simulink model "propagator_mess"  (R2023b)
settings: Solver=VariableStepAuto  StartTime=0.0  StopTime=tf  RelTol=1e-10  AbsTol=1e-10
undefined symbols (not defined in the file or in its folder): mass, thrust, thrustingThreshold
libraries: vrlib x3, simulink x1, aerolibsatdyn x1, aerolibutil x1
settings Model: SimulationMode=rapid-accelerator  Creator=miqui  LastModifiedBy=miqui

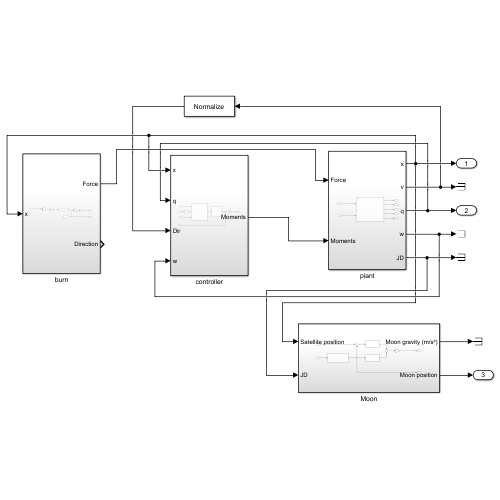
[thumbnail: Simulink's stored preview of the top-level diagram]
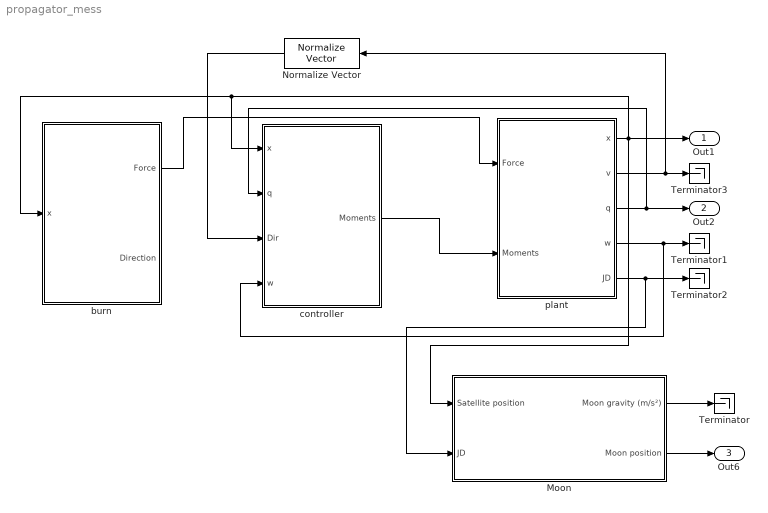
== system propagator_mess ==
  Moon : Subsystem
  Normalize Vector : vrlib/Utilities/Normalize Vector  maxzero=0
  Terminator{,1..3} (4 alike) : Terminator
  burn : Subsystem
  controller : Subsystem
  plant : Subsystem
  Out1 : Outport
  Out2 : Outport  Port=2
  Out6 : Outport  Port=3
  wires:
  plant/1(x) -> controller/1(x), burn/1(x), Moon/1(Satellite position), Out1/1
  plant/2(v) -> Normalize Vector/1, Terminator3/1
  plant/3(q) -> Out2/1, controller/2(q)
  plant/4(w) -> Terminator1/1, controller/4(w)
  plant/5(JD) -> Terminator2/1, Moon/2(JD)
  Moon/1(Moon gravity (m/s²)) -> Terminator/1
  Moon/2(Moon position) -> Out6/1
  Normalize Vector/1 -> controller/3(Dir)
  controller/1(Moments) -> plant/2(Moments)
  burn/1(Force) -> plant/1(Force)

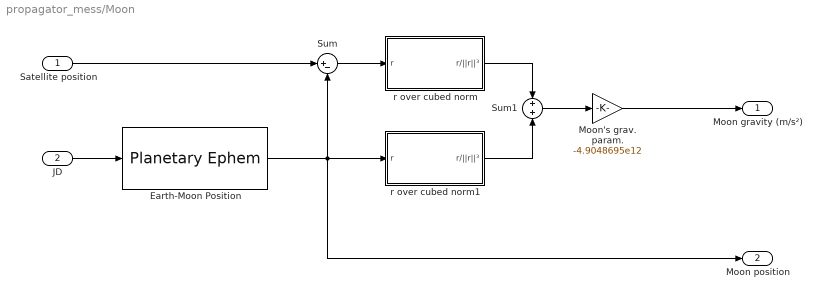
== system propagator_mess/Moon ==
  Satellite position : Inport
  JD : Inport  Port=2
  Earth-Moon Position : PlanetaryEphem  units=m,m/s  useDateRange=on  outputVelocity=off
  Moon's grav. param. : Gain  Gain=-4.9048695e12
  Sum : Sum  Inputs=|+-
  Sum1 : Sum
  r over cubed norm : Subsystem
  r over cubed norm1 : Subsystem
  Moon gravity (m/s²) : Outport
  Moon position : Outport  Port=2
  wires:
  JD/1 -> Earth-Moon Position/1
  Satellite position/1 -> Sum/1
  Earth-Moon Position/1 -> Moon position/1, r over cubed norm1/1(r), Sum/2
  Sum/1 -> r over cubed norm/1(r)
  Sum1/1 -> Moon's grav. param./1
  Moon's grav. param./1 -> Moon gravity (m/s²)/1
  r over cubed norm/1(r/||r||³) -> Sum1/1
  r over cubed norm1/1(r/||r||³) -> Sum1/2

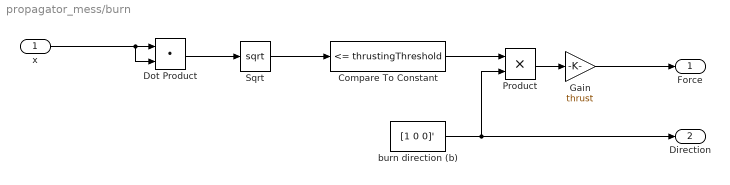
== system propagator_mess/burn ==
  x : Inport
  Compare To Constant : simulink/Logic and Bit Operations/Compare To Constant  relop=<=  const=thrustingThreshold  OutDataTypeStr=boolean
  Dot Product : DotProduct  OutDataTypeStr=Inherit: Inherit via internal rule
  Gain : Gain  Gain=thrust
  Product : Product
  Sqrt : Sqrt
  burn direction (b) : Constant  Value=[1 0 0]'
  Force : Outport
  Direction : Outport  Port=2
  wires:
  Dot Product/1 -> Sqrt/1
  Sqrt/1 -> Compare To Constant/1
  x/1 -> Dot Product/2, Dot Product/1
  burn direction (b)/1 -> Direction/1, Product/2
  Gain/1 -> Force/1
  Compare To Constant/1 -> Product/1
  Product/1 -> Gain/1

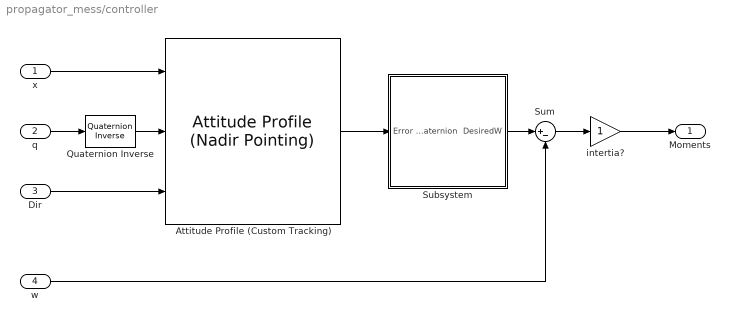
== system propagator_mess/controller ==
  x : Inport
  q : Inport  Port=2
  Dir : Inport  Port=3
  w : Inport  Port=4
  Attitude Profile (Custom Tracking) : aerolibsatdyn/Attitude Profile (Nadir Pointing)  outputError=on  outputFinalAttitude=off  portFrame=ICRF  pointingMode=Custom  celestialTarget=Sun  tunablePointing=off  primaryAlignmentSrc=Dialog  primaryAlignment=[1 0 0]  secondaryAlignmentSrc=Dialog  secondaryAlignment=[0 0 1]  constraintFrame=ICRF  primaryConstraintSrc=Port  primaryConstraint=[1 0 0]  secondaryConstraintSrc=Dialog  secondaryConstraint=[0 0 1]
      settings: LibrarySourceBlock=|
      | aerolibsatdyn/Attitude Profile
      | (Sun Tracking)
  Quaternion Inverse : aerolibutil/Quaternion Inverse
  Subsystem : Subsystem
  Sum : Sum  Inputs=|+-
  intertia? : Gain
  Moments : Outport
  wires:
  intertia?/1 -> Moments/1
  x/1 -> Attitude Profile (Custom Tracking)/1
  q/1 -> Quaternion Inverse/1
  Quaternion Inverse/1 -> Attitude Profile (Custom Tracking)/2
  Sum/1 -> intertia?/1
  w/1 -> Sum/2
  Attitude Profile (Custom Tracking)/1 -> Subsystem/1(Error quaternion)
  Subsystem/1(DesiredW) -> Sum/1
  Dir/1 -> Attitude Profile (Custom Tracking)/3

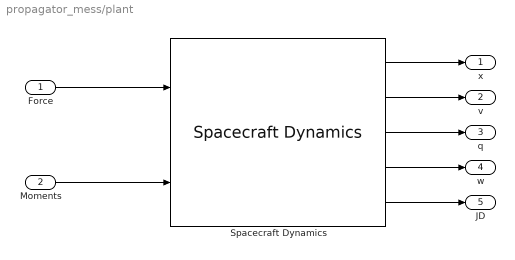
== system propagator_mess/plant ==
  Force : Inport
  Moments : Inport  Port=2
  Spacecraft Dynamics : SpacecraftDynamics  mass=mass  inertia=[1, 0, 0; 0, 1, 0; 0, 0, 1]*mass  useMassFlowRelativeVelocity=on  semiMajorAxis=sma  eccentricity=ecc  inclination=inc  raan=RAAN  argPeriapsis=aop  trueAnomaly=true_an  gravityModel=Point-mass  useEOPs=off
  x : Outport
  v : Outport  Port=2
  q : Outport  Port=3
  w : Outport  Port=4
  JD : Outport  Port=5
  wires:
  Spacecraft Dynamics/5 -> JD/1
  Spacecraft Dynamics/1 -> x/1
  Force/1 -> Spacecraft Dynamics/1
  Moments/1 -> Spacecraft Dynamics/2
  Spacecraft Dynamics/4 -> w/1
  Spacecraft Dynamics/2 -> v/1
  Spacecraft Dynamics/3 -> q/1

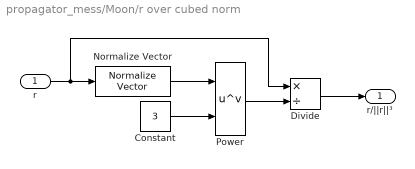
== system propagator_mess/Moon/r over cubed norm ==
  r : Inport
  Constant : Constant  Value=3
  Divide : Product  Inputs=*/
  Normalize Vector : vrlib/Utilities/Normalize Vector  maxzero=0
  Power : Math  Operator=pow
  r/||r||³ : Outport
  wires:
  r/1 -> Divide/1, Normalize Vector/1
  Normalize Vector/1 -> Power/1
  Constant/1 -> Power/2
  Power/1 -> Divide/2
  Divide/1 -> r/||r||³/1

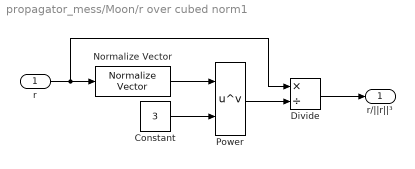
== system propagator_mess/Moon/r over cubed norm1 ==
  r : Inport
  Constant : Constant  Value=3
  Divide : Product  Inputs=*/
  Normalize Vector : vrlib/Utilities/Normalize Vector  maxzero=0
  Power : Math  Operator=pow
  r/||r||³ : Outport
  wires:
  r/1 -> Divide/1, Normalize Vector/1
  Normalize Vector/1 -> Power/1
  Constant/1 -> Power/2
  Power/1 -> Divide/2
  Divide/1 -> r/||r||³/1

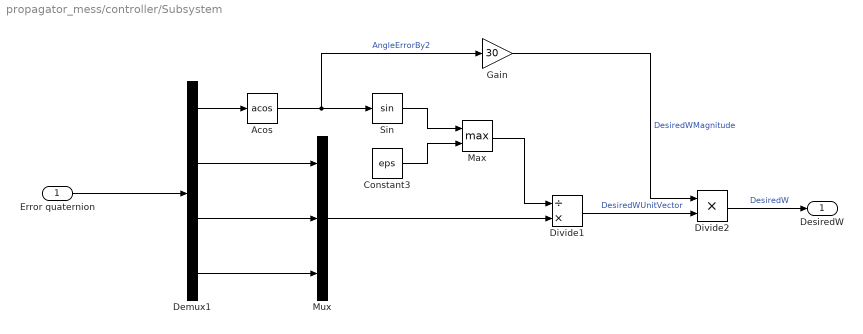
== system propagator_mess/controller/Subsystem ==
  Error quaternion : Inport
  Acos : Trigonometry  Operator=acos
  Constant3 : Constant  Value=eps
  Demux1 : Demux
  Divide1 : Product  Inputs=/*
  Divide2 : Product  Inputs=**
  Gain : Gain  Gain=30
  Max : MinMax  Function=max  Inputs=2
  Mux : Mux  Inputs=3
  Sin : Trigonometry
  DesiredW : Outport
  wires:
  Error quaternion/1 -> Demux1/1
  Gain/1 -> Divide2/1  "DesiredWMagnitude"
  Demux1/2 -> Mux/1
  Demux1/1 -> Acos/1
  Acos/1 -> Sin/1, Gain/1  "AngleErrorBy2"
  Mux/1 -> Divide1/2
  Divide2/1 -> DesiredW/1  "DesiredW"
  Constant3/1 -> Max/2
  Demux1/3 -> Mux/2
  Max/1 -> Divide1/1
  Demux1/4 -> Mux/3
  Sin/1 -> Max/1
  Divide1/1 -> Divide2/2  "DesiredWUnitVector"
